simulink model "Boost_Non_Ideal_Linear_Model"  (R2022b)
settings: Solver=VariableStepAuto  StartTime=0.0  StopTime=0.02  RelTol=1e-3
values from neighbouring files (symbols this model uses):
  C = 1e-3    (= 0.001)    [Boost_Converter_Parameters.m]
  Dnom = 0.55    [Boost_Converter_Parameters.m]
  fS = 10^5    (= 100000)    [Boost_Converter_Parameters.m]
  L = 100e-6    (= 0.0001)    [Boost_Converter_Parameters.m]
  RL = 4.5    [Boost_Converter_Parameters.m]
  Vinnom = 24    [Boost_Converter_Parameters.m]
settings Model: Creator=YESHIWAS  LastModifiedBy=YESHIWAS
settings DataIOCC: ReturnWorkspaceOutputs=off

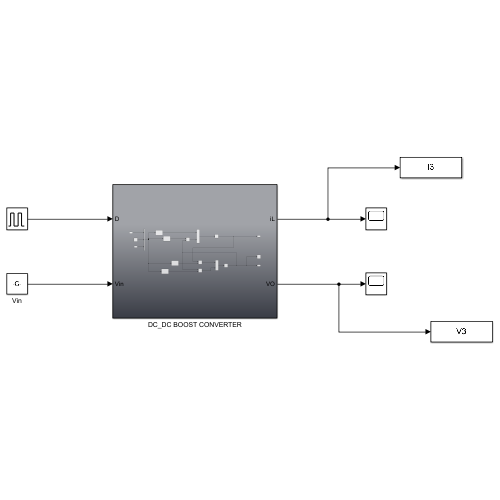
[thumbnail: Simulink's stored preview of the top-level diagram]
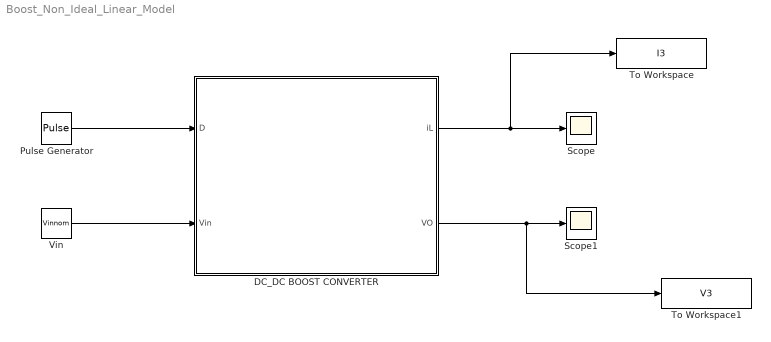
== system Boost_Non_Ideal_Linear_Model ==
  DC_DC BOOST CONVERTER : Subsystem
  Pulse Generator : DiscretePulseGenerator  PulseType=Time based  Period=1/fS  PulseWidth=Dnom*100
  Scope : Scope
  Scope1 : Scope
  To Workspace : ToWorkspace  VariableName=I3  SaveFormat=Structure With Time  SampleTime=-1
  To Workspace1 : ToWorkspace  VariableName=V3  SaveFormat=Structure With Time  SampleTime=-1
  Vin : Constant  Value=Vinnom
  wires:
  Pulse Generator/1 -> DC_DC BOOST CONVERTER/1(D)
  Vin/1 -> DC_DC BOOST CONVERTER/2(Vin)
  DC_DC BOOST CONVERTER/2(VO) -> To Workspace1/1, Scope1/1
  DC_DC BOOST CONVERTER/1(iL) -> To Workspace/1, Scope/1

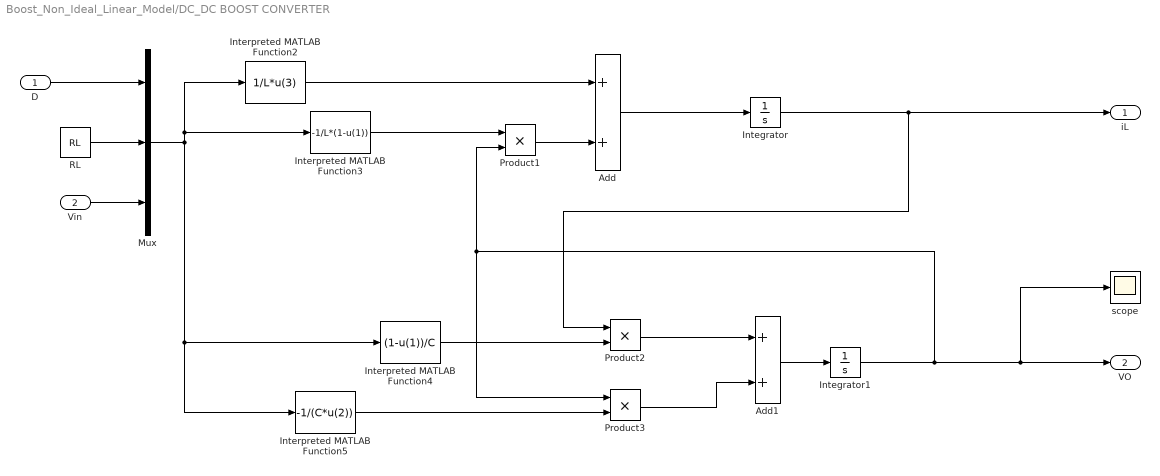
== system Boost_Non_Ideal_Linear_Model/DC_DC BOOST CONVERTER ==
  D : Inport
  Vin : Inport  Port=2
  Add : Sum
  Add1 : Sum
  Integrator : Integrator
  Integrator1 : Integrator
  Interpreted MATLAB Function2 : MATLABFcn  MATLABFcn=1/L*u(3)
  Interpreted MATLAB Function3 : MATLABFcn  MATLABFcn=-1/L*(1-u(1))
  Interpreted MATLAB Function4 : MATLABFcn  MATLABFcn=(1-u(1))/C
  Interpreted MATLAB Function5 : MATLABFcn  MATLABFcn=-1/(C*u(2))
  Mux : Mux  Inputs=3
  Product1 : Product
  Product2 : Product
  Product3 : Product
  RL : Constant  Value=RL
  scope : Scope
  iL : Outport
  VO : Outport  Port=2
  wires:
  Integrator/1 -> Product2/1, iL/1
  Add/1 -> Integrator/1
  Add1/1 -> Integrator1/1
  Interpreted MATLAB Function3/1 -> Product1/1
  Interpreted MATLAB Function2/1 -> Add/1
  Mux/1 -> Interpreted MATLAB Function3/1, Interpreted MATLAB Function2/1, Interpreted MATLAB Function4/1, Interpreted MATLAB Function5/1
  Interpreted MATLAB Function4/1 -> Product2/2
  Interpreted MATLAB Function5/1 -> Product3/2
  Product3/1 -> Add1/2
  Product2/1 -> Add1/1
  D/1 -> Mux/1
  RL/1 -> Mux/2
  Vin/1 -> Mux/3
  Integrator1/1 -> VO/1, scope/1, Product3/1, Product1/2
  Product1/1 -> Add/2
